simulink model "mpc_blueboat"  (R2024a)
settings: Solver=VariableStepAuto  StartTime=0.0  StopTime=20  RelTol=1e-3
libraries: sharedutil x6, aerolibutil x1, mpclib x1
settings Model: Creator=cdsouza
settings SolverCC: AlgebraicLoopSolver=TrustRegion
settings DataIOCC: ReturnWorkspaceOutputs=off
settings DebuggingCC: UnconnectedInputMsg=warning  UnconnectedOutputMsg=warning  UnconnectedLineMsg=warning  ArithmeticOperatorsInVariantConditions=warning
settings ModelReferenceCC: EnableRefExpFcnMdlSchedulingChecks=on
settings SFSimCC: CustomCodeUndefinedFunction=UseInterfaceOnly
settings RTWCC: GPUComputeCapability=3.5

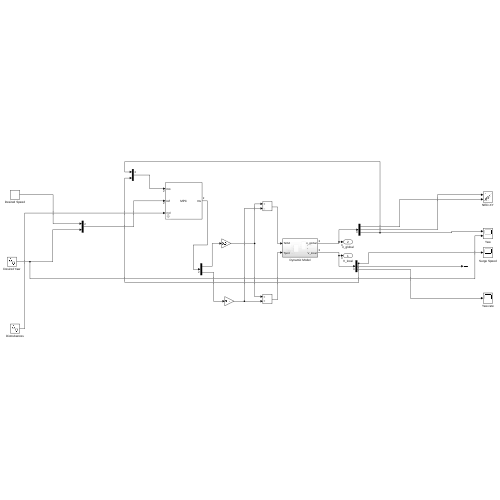
[thumbnail: Simulink's stored preview of the top-level diagram]
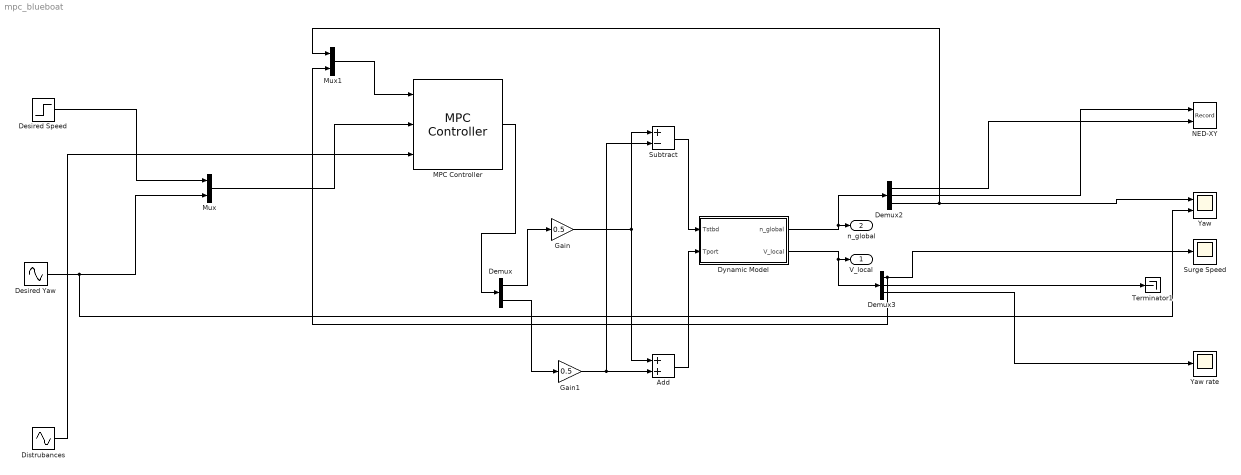
== system mpc_blueboat ==
  Add : Sum
  Demux : Demux  Outputs=2
  Demux2 : Demux  Outputs=3
  Demux3 : Demux  Outputs=3
  Desired Speed : Step  Time=2  SampleTime=0
  Desired Yaw : Sin  Amplitude=5  Frequency=0.5  SampleTime=0
  Distrubances : Sin  Amplitude=0.001  Frequency=0.5  SampleTime=0
  Dynamic Model : Subsystem
  Gain : Gain  Gain=0.5
  Gain1 : Gain  Gain=0.5
  MPC Controller : mpclib/MPC Controller  SCDEnableBlockLinearizationSpecification=on  mpcobj=mpc1  is_multiple=0  enable_value=0  return_u0=off  updateMPCinCallerWorkspace=on  md_inport=on  mv_inport=off  uref_inport=off  return_cost=off  return_mvseq=off  return_qpstatus=off  return_xseq=off  return_state=off  return_ovseq=off  state_inport=off  umin_inport=off  umax_inport=off  ymin_inport=off  ymax_inport=off  cc_inport=off  ywt_inport=off  uwt_inport=off  duwt_inport=off  rhoeps_inport=off  pm_inport=off  MaximumP=10  HorizonChoice=FixedHorizon  n_ts=0.1  n_p=20  n_mv=2  n_md=1  n_ud=0  n_mo=2  n_uo=0  BlockDataType=double  SampleTimeInherited=off  switch_inport=off
  Mux : Mux  Inputs=2
  Mux1 : Mux  Inputs=2
  NED-XY : Record  FileSettingsInternal="{\"entries\":[{\"content\":{\"excelSettings\":{\"content\":{},\"type\":\"Streamout.ExcelSettings\"}},\"type\":\"Streamout.FileSettingStorage\",\"uuid\":\"\"}],\"packageUris\":[\"http:\\/\\/schema.mathworks.com\\/mf0\\/streamout_blocks\\/R2020a\"],\"version\":\"1.0\"}"  Layout=[1 1]  SignalsInternal="{\"entries\":[{\"content\":{\"signals\":[{\"content\":{\"blockPath\":[],\"dimensions\":[1],\"domain\":\"\",\"lineColor\":\"#a2142f\",\"plots\":[ 1 ],\"port\":1,\"sid\":[\"\"],\"signalID\":1,\"signalName\":\"Demux2:2\"},\"type\":\"RecordBlkView.Signal\",\"uuid\":\"\"},{\"content\":{\"blockPath\":[],\"dimensions\":[1],\"domain\":\"\",\"lineColor\":\"#139fff\",\"plots\":[ 1 ],\"port\":2,\"sid\":[\"\"],\"signalID\":2,\"signalName\":\"Demux2:1\"},\"type\":\"RecordBlkView.Signal\",\"uuid\":\"\"},{\"content\":{\"blockPath\":[],\"dimensions\":[3],\"domain\":\"\",\"hasChildren\":true,\"lineColor\":\"#edb120\",\"lineWidth\":2,\"port\":1,\"sid\":[\"\"],\"signalID\":3},\"type\":\"RecordBlkView.Signal\",\"uuid\":\"\"},{\"content\":{\"blockPath\":[],\"channel\":[1],\"dimensions\":[3],\"domain\":\"\",\"lineColor\":\"#b746ff\",\"lineWidth\":2,\"parentID\":3,\"port\":1,\"sid\":[\"\"],\"signalID\":4},\"type\":\"RecordBlkView.Signal\",\"uuid\":\"\"},{\"content\":{\"blockPath\":[],\"dimensions\":[3],\"domain\":\"\",\"hasChildren\":true,\"lineColor\":\"#77ac30\",\"lineWidth\":2,\"port\":1,\"sid\":[\"\"],\"signalID\":5},\"type\":\"RecordBlkView.Signal\",\"uuid\":\"\"},{\"content\":{\"blockPath\":[],\"channel\":[1],\"dimensions\":[3],\"domain\":\"\",\"lineColor\":\"#ff13a6\",\"lineWidth\":2,\"parentID\":5,\"port\":1,\"sid\":[\"\"],\"signalID\":6},\"type\":\"RecordBlkView.Signal\",\"uuid\":\"\"},{\"content\":{\"blockPath\":[],\"dimensions\":[1],\"domain\":\"\",\"hasChildren\":true,\"lineColor\":\"#a2142f\",\"lineWidth\":2,\"port\":1,\"sid\":[\"\"],\"signalID\":7,\"signalName\":\"HydrodynamicCoefficients\"},\"type\":\"RecordBlkView.Signal\",\"uuid\":\"\"},{\"content\":{\"blockPath\":[],\"dimensions\":[1],\"domain\":\"\",\"leafPath\":\"HydrodynamicCoefficients.X_u_dot\",\"lineColor\":\"#139fff\",\"lineWidth\":2,\"parentID\":7,\"port\":1,\"sid\":[\"\"],\"signalID\":8,\"signalName\":\"HydrodynamicCoefficients.X_u_dot\"},\"type\":\"RecordBlkView.Signal\",\"uuid\":\"\"},{\"content\":{\"blockPath\":[],\"dimensions\":[1],\"domain\":\"\",\"leafPath\":\"HydrodynamicCoefficients.Y_v_dot\",\"lineColor\":\"#ff6929\",\"lineWidth\":2,\"parentID\":7,\"port\":1,\"sid\":[\"\"],\"signalID\":9,\"signalName\":\"HydrodynamicCoefficients.Y_v_dot\"},\"type\":\"RecordBlkView.Signal\",\"uuid\":\"\"},{\"content\":{\"blockPath\":[],\"dimensions\":[1],\"domain\":\"\",\"leafPath\":\"HydrodynamicCoefficients.Y_r_dot\",\"lineColor\":\"#b746ff\",\"lineWidth\":2,\"parentID\":7,\"port\":1,\"sid\":[\"\"],\"signalID\":10,\"signalName\":\"HydrodynamicCoefficients.Y_r_dot\"},\"type\":\"RecordBlkView.Signal\",\"uuid\":\"\"},{\"content\":{\"blockPath\":[],\"dimensions\":[1],\"domain\":\"\",\"leafPath\":\"HydrodynamicCoefficients.N_v_dot\",\"lineColor\":\"#64d413\",\"lineWidth\":2,\"parentID\":7,\"port\":1,\"sid\":[\"\"],\"signalID\":11,\"signalName\":\"HydrodynamicCoefficients.N_v_dot\"},\"type\":\"RecordBlkView.Signal\",\"uuid\":\"\"},{\"content\":{\"blockPath\":[],\"dimensions\":[1],\"domain\":\"\",\"leafPath\":\"HydrodynamicCoefficients.N_r_dot\",\"lineColor\":\"#ff13a6\",\"lineWidth\":2,\"parentID\":7,\"port\":1,\"sid\":[\"\"],\"signalID\":12,\"signalName\":\"HydrodynamicCoefficients.N_r_dot\"},\"type\":\"RecordBlkView.Signal\",\"uuid\":\"\"},{\"content\":{\"blockPath\":[],\"dimensions\":[1],\"domain\":\"\",\"leafPath\":\"HydrodynamicCoefficients.X_u\",\"lineColor\":\"#fe330a\",\"lineWidth\":2,\"parentID\":7,\"port\":1,\"sid\":[\"\"],\"signalID\":13,\"signalName\":\"HydrodynamicCoefficients.X_u\"},\"type\":\"RecordBlkView.Signal\",\"uuid\":\"\"},{\"content\":{\"blockPath\":[],\"dimensions\":[1],\"domain\":\"\",\"leafPath\":\"HydrodynamicCoefficients.X_u_u_\",\"lineColor\":\"#22b573\",\"lineWidth\":2,\"parentID\":7,\"port\":1,\"sid\":[\"\"],\"signalID\":14,\"signalName\":\"HydrodynamicCoefficients.X_u_u_\"},\"type\":\"RecordBlkView.Signal\",\"uuid\":\"\"},{\"content\":{\"blockPath\":[],\"dimensions\":[1],\"domain\":\"\",\"leafPath\":\"HydrodynamicCoefficients.Y_v_v_\",\"lineColor\":\"#0072bd\",\"lineWidth\":2,\"parentID\":7,\"port\":1,\"sid\":[\"\"],\"signalID\":15,\"signalName\":\"HydrodynamicCoefficients.Y_v_v_\"},\"type\":\"RecordBlkView.Signal\",\"uuid\":\"\"},{\"content\":{\"blockPath\":[],\"dimensions\":[1],\"domain\":\"\",\"leafPath\":\"HydrodynamicCoefficients.Y_v_r_\",\"lineColor\":\"#d95319\",\"lineWidth\":2,\"parentID\":7,\"port\":1,\"sid\":[\"\"],\"signalID\":16,\"signalName\":\"HydrodynamicCoefficients.Y_v_r_\"},\"type\":\"RecordBlkView.Signal\",\"uuid\":\"\"},{\"content\":{\"blockPath\":[],\"dimensions\":[1],\"domain\":\"\",\"leafPath\":\"HydrodynamicCoefficients.Y_v\",\"lineColor\":\"#edb120\",\"lineWidth\":2,\"parentID\":7,\"port\":1,\"sid\":[\"\"],\"signalID\":17,\"signalName\":\"HydrodynamicCoefficients.Y_v\"},\"type\":\"RecordBlkView.Signal\",\"uuid\":\"\"},{\"content\":{\"blockPath\":[],\"dimensions\":[1],\"domain\":\"\",\"leafPath\":\"HydrodynamicCoefficients.Y_r_v_\",\"lineColor\":\"#7e2f8e\",\"lineWidth\":2,\"parentID\":7,\"port\":1,\"sid\":[\"\"],\"signalID\":18,\"signalName\":\"HydrodynamicCoefficients.Y_r_v_\"},\"type\":\"RecordBlkView.Signal\",\"uuid\":\"\"},{\"content\":{\"blockPath\":[],\"dimensions\":[1],\"domain\":\"\",\"leafPath\":\"HydrodynamicCoefficients.Y_r_r_\",\"lineColor\":\"#77ac30\",\"lineWidth\":2,\"parentID\":7,\"port\":1,\"sid\":[\"\"],\"signalID\":19,\"signalName\":\"HydrodynamicCoefficients.Y_r_r_\"},\"type\":\"RecordBlkView.Signal\",\"uuid\":\"\"},{\"content\":{\"blockPath\":[],\"dimensions\":[1],\"domain\":\"\",\"leafPath\":\"HydrodynamicCoefficients.Y_r\",\"lineColor\":\"#4dbeee\",\"lineWidth\":2,\"parentID\":7,\"port\":1,\"sid\":[\"\"],\"signalID\":20,\"signalName\":\"HydrodynamicCoefficients.Y_r\"},\"type\":\"RecordBlkView.Signal\",\"uuid\":\"\"},{\"content\":{\"blockPath\":[],\"dimensions\":[1],\"domain\":\"\",\"leafPath\":\"HydrodynamicCoefficients.N_v_v_\",\"lineColor\":\"#a2142f\",\"lineWidth\":2,\"parentID\":7,\"port\":1,\"sid\":[\"\"],\"signalID\":21,\"signalName\":\"HydrodynamicCoefficients.N_v_v_\"},\"type\":\"RecordBlkView.Signal\",\"uuid\":\"\"},{\"content\":{\"blockPath\":[],\"dimensions\":[1],\"domain\":\"\",\"leafPath\":\"HydrodynamicCoefficients.N_v\",\"lineColor\":\"#139fff\",\"lineWidth\":2,\"parentID\":7,\"port\":1,\"sid\":[\"\"],\"signalID\":22,\"signalName\":\"HydrodynamicCoefficients.N_v\"},\"type\":\"RecordBlkView.Signal\",\"uuid\":\"\"},{\"content\":{\"blockPath\":[],\"dimensions\":[1],\"domain\":\"\",\"leafPath\":\"HydrodynamicCoefficients.N_v_r_\",\"lineColor\":\"#ff6929\",\"lineWidth\":2,\"parentID\":7,\"port\":1,\"sid\":[\"\"],\"signalID\":23,\"signalName\":\"HydrodynamicCoefficients.N_v_r_\"},\"type\":\"RecordBlkView.Signal\",\"uuid\":\"\"},{\"content\":{\"blockPath\":[],\"dimensions\":[1],\"domain\":\"\",\"leafPath\":\"HydrodynamicCoefficients.N_r_v_\",\"lineColor\":\"#b746ff\",\"lineWidth\":2,\"parentID\":7,\"port\":1,\"sid\":[\"\"],\"signalID\":24,\"signalName\":\"HydrodynamicCoefficients.N_r_v_\"},\"type\":\"RecordBlkView.Signal\",\"uuid\":\"\"},{\"content\":{\"blockPath\":[],\"dimensions\":[1],\"domain\":\"\",\"leafPath\":\"HydrodynamicCoefficients.N_r\",\"lineColor\":\"#64d413\",\"lineWidth\":2,\"parentID\":7,\"port\":1,\"sid\":[\"\"],\"signalID\":25,\"signalName\":\"HydrodynamicCoefficients.N_r\"},\"type\":\"RecordBlkView.Signal\",\"uuid\":\"\"},{\"content\":{\"blockPath\":[],\"dimensions\":[1],\"domain\":\"\",\"leafPath\":\"HydrodynamicCoefficients.N_r_r_\",\"lineColor\":\"#ff13a6\",\"lineWidth\":2,\"parentID\":7,\"port\":1,\"sid\":[\"\"],\"signalID\":26,\"signalName\":\"HydrodynamicCoefficients.N_r_r_\"},\"type\":\"RecordBlkView.Signal\",\"uuid\":\"\"},{\"content\":{\"blockPath\":[],\"channel\":[2],\"dimensions\":[3],\"domain\":\"\",\"lineColor\":\"#edb120\",\"lineWidth\":2,\"parentID\":3,\"port\":1,\"sid\":[\"\"],\"signalID\":27},\"type\":\"RecordBlkView.Signal\",\"uuid\":\"\"},{\"content\":{\"blockPath\":[],\"channel\":[3],\"dimensions\":[3],\"domain\":\"\",\"lineColor\":\"#7e2f8e\",\"lineWidth\":2,\"parentID\":3,\"port\":1,\"sid\":[\"\"],\"signalID\":28},\"type\":\"RecordBlkView.Signal\",\"uuid\":\"\"},{\"content\":{\"blockPath\":[],\"channel\":[2],\"dimensions\":[3],\"domain\":\"\",\"lineColor\":\"#77ac30\",\"lineWidth\":2,\"parentID\":5,\"port\":1,\"sid\":[\"\"],\"signalID\":29},\"type\":\"RecordBlkView.Signal\",\"uuid\":\"\"},{\"content\":{\"blockPath\":[],\"channel\":[3],\"dimensions\":[3],\"domain\":\"\",\"lineColor\":\"#4dbeee\",\"lineWidth\":2,\"parentID\":5,\"port\":1,\"sid\":[\"\"],\"signalID\":30},\"type\":\"RecordBlkView.Signal\",\"uuid\":\"\"}]},\"type\":\"RecordBlkView.InputSignals\",\"uuid\":\"\"}],\"packageUris\":[\"http:\\/\\/schema.mathworks.com\\/mf0\\/streamout_blocks\\/R2020a\"],\"version\":\"1.0\"}"  VisualizationBindings="{\"xyplotplugin\":{\"info\":[{\"series\":[{\"bindingParametersList\":[{\"parameter\":\"X-Axis\",\"signalID\":1,\"signalName\":\"Demux2:2\"},{\"parameter\":\"Y-Axis\",\"signalID\":2,\"signalName\":\"Demux2:1\"}],\"seriesID\":0}],\"subplotID\":1}]}}"  CompatibilityTag=XY  st=-1
  Subtract : Sum  Inputs=+-
  Surge Speed : Scope
  Terminator1 : Terminator
  Yaw : Scope  NumInputPorts=2
  Yaw rate : Scope
  V_local : Outport  VectorParamsAs1DForOutWhenUnconnected=off
  n_global : Outport  Port=2  VectorParamsAs1DForOutWhenUnconnected=off
  wires:
  Dynamic Model/1(n_global) -> Demux2/1, n_global/1
  Demux2/2 -> NED-XY/1
  Demux2/1 -> NED-XY/2
  Demux3/1 -> Mux1/2, Surge Speed/1
  Demux3/3 -> Yaw rate/1
  Dynamic Model/2(V_local) -> Demux3/1, V_local/1
  Demux2/3 -> Mux1/1, Yaw/1
  Demux3/2 -> Terminator1/1
  Desired Yaw/1 -> Yaw/2, Mux/2
  Gain/1 -> Subtract/1, Add/1
  Gain1/1 -> Add/2, Subtract/2
  Add/1 -> Dynamic Model/2(Tport)
  Subtract/1 -> Dynamic Model/1(Tstbd)
  Desired Speed/1 -> Mux/1
  Mux/1 -> MPC Controller/2
  Distrubances/1 -> MPC Controller/3
  Demux/2 -> Gain1/1
  Demux/1 -> Gain/1
  MPC Controller/1 -> Demux/1
  Mux1/1 -> MPC Controller/1

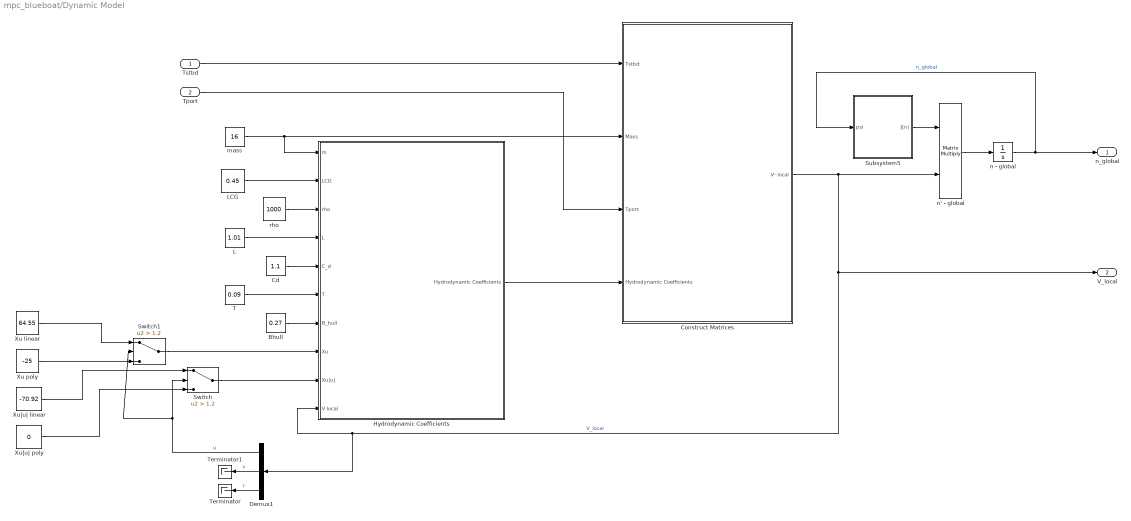
== system mpc_blueboat/Dynamic Model ==
  Tstbd : Inport
  Tport : Inport  Port=2
  "Bhull " : Constant  Value=0.27
  Cd : Constant  Value=1.1
  Construct Matrices : Subsystem
  Demux1 : Demux  Outputs=3
  Hydrodynamic Coefficients : Subsystem
  L : Constant  Value=1.01
  LCG : Constant  Value=0.45
  Subsystem5 : Subsystem
  Switch : Switch  Criteria=u2 > Threshold  Threshold=1.2  SaturateOnIntegerOverflow=off  InputSameDT=off
  Switch1 : Switch  Criteria=u2 > Threshold  Threshold=1.2  SaturateOnIntegerOverflow=off  InputSameDT=off
  T : Constant  Value=0.09
  Terminator : Terminator
  Terminator1 : Terminator
  Xu linear : Constant  Value=64.55
  Xu poly : Constant  Value=-25
  Xu|u| linear : Constant  Value=-70.92
  Xu|u| poly : Constant  Value=0
  mass : Constant  Value=16
  n - global : Integrator  InitialCondition=[0 0 0]
  n' - global : Product  Multiplication=Matrix(*)
  rho : Constant  Value=1000
  n_global : Outport  VectorParamsAs1DForOutWhenUnconnected=off
  V_local : Outport  Port=2  VectorParamsAs1DForOutWhenUnconnected=off
  wires:
  n - global/1 -> n_global/1, Subsystem5/1(psi)  "n_global"
  Cd/1 -> Hydrodynamic Coefficients/5(C_d)
  Construct Matrices/1(V- local) -> Demux1/1, Hydrodynamic Coefficients/10(V local), V_local/1, n' - global/2  "V_local"
  n' - global/1 -> n - global/1
  Subsystem5/1(J(n)) -> n' - global/1
  rho/1 -> Hydrodynamic Coefficients/3(rho)
  L/1 -> Hydrodynamic Coefficients/4(L)
  Tport/1 -> Construct Matrices/3(Tport)
  Tstbd/1 -> Construct Matrices/1(Tstbd)
  mass/1 -> Hydrodynamic Coefficients/1(m), Construct Matrices/2("Mass ")
  Hydrodynamic Coefficients/1("Hydrodynamic Coefficients ") -> Construct Matrices/4(Hydrodynamic Coefficients)
  T/1 -> Hydrodynamic Coefficients/6(T)
  "Bhull "/1 -> Hydrodynamic Coefficients/7(B_hull)
  Switch/1 -> Hydrodynamic Coefficients/9(Xu|u|)
  LCG/1 -> Hydrodynamic Coefficients/2(LCG)
  Demux1/1 -> Switch1/2, Switch/2  "u"
  Xu|u| poly/1 -> Switch/3
  Xu|u| linear/1 -> Switch/1
  Switch1/1 -> Hydrodynamic Coefficients/8(Xu)
  Xu poly/1 -> Switch1/3
  Xu linear/1 -> Switch1/1
  Demux1/3 -> Terminator/1  "r"
  Demux1/2 -> Terminator1/1  "v"

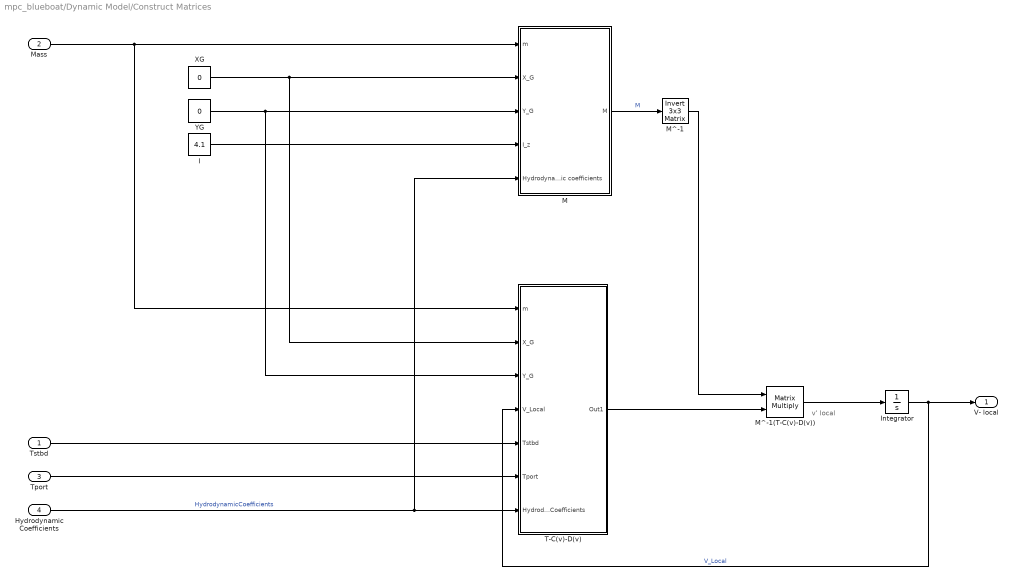
== system mpc_blueboat/Dynamic Model/Construct Matrices ==
  note: v' local
  Tstbd : Inport
  "Mass " : Inport  Port=2
  Tport : Inport  Port=3
  Hydrodynamic Coefficients : Inport  Port=4
  I : Constant  Value=4.1
  Integrator : Integrator
  M : Subsystem
  M^-1 : aerolibutil/Invert  3x3 Matrix
  M^-1(T-C(v)-D(v)) : Product  Multiplication=Matrix(*)
  T-C(v)-D(v) : Subsystem
  XG : Constant  Value=0
  YG : Constant  Value=0
  V- local : Outport  VectorParamsAs1DForOutWhenUnconnected=off
  wires:
  M/1(M) -> M^-1/1  "M"
  Integrator/1 -> V- local/1, T-C(v)-D(v)/4(V_Local)  "V_Local"
  M^-1(T-C(v)-D(v))/1 -> Integrator/1
  I/1 -> M/4(I_z)
  M^-1/1 -> M^-1(T-C(v)-D(v))/1
  Hydrodynamic Coefficients/1 -> M/5(Hydrodynamic coefficients), T-C(v)-D(v)/7(HydrodynamicCoefficients)  "HydrodynamicCoefficients"
  YG/1 -> T-C(v)-D(v)/3(Y_G), M/3(Y_G)
  "Mass "/1 -> T-C(v)-D(v)/1(m), M/1(m)
  XG/1 -> T-C(v)-D(v)/2(X_G), M/2(X_G)
  Tstbd/1 -> T-C(v)-D(v)/5(Tstbd)
  Tport/1 -> T-C(v)-D(v)/6(Tport)
  T-C(v)-D(v)/1(Out1) -> M^-1(T-C(v)-D(v))/2

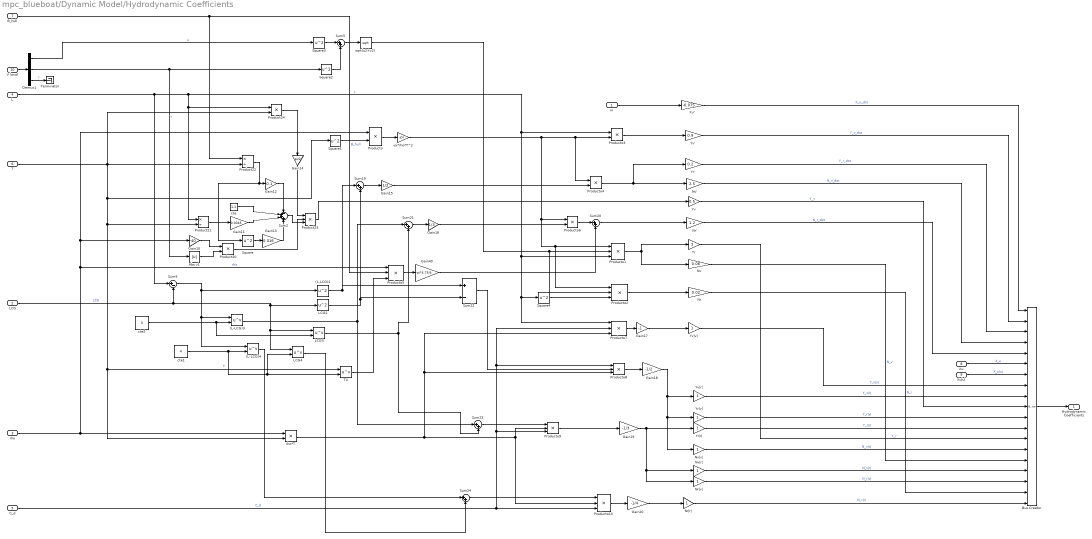
== system mpc_blueboat/Dynamic Model/Hydrodynamic Coefficients ==
  m : Inport
  LCG : Inport  Port=2
  rho : Inport  Port=3
  L : Inport  Port=4
  C_d : Inport  Port=5
  T : Inport  Port=6
  B_hull : Inport  Port=7
  Xu : Inport  Port=8
  Xu|u| : Inport  Port=9
  V local : Inport  Port=10
  (L-LCG)2 : Math  Operator=square  SignedPower=on
  (L-LCG)3 : Math  Operator=pow  SignedPower=on
  (L-LCG)4 : Math  Operator=pow  SignedPower=on
  -pi*rho*T^2 : Gain  Gain=-pi
  Abs v1 : Abs  SaturateOnIntegerOverflow=off
  Bus Creator : BusCreator  Inputs=19
  Demux1 : Demux  Outputs=3
  Gain10 : Gain  Gain=-40
  Gain11 : Gain  Gain=0.0045
  Gain12 : Gain  Gain=0.1
  Gain13 : Gain  Gain=0.016
  Gain14 : Gain  Gain=pi/2
  Gain15 : Gain  Gain=1/2
  Gain16 : Gain  Gain=1/3
  Gain17 : Gain  Gain=-1
  Gain18 : Gain  Gain=-1/2
  Gain19 : Gain  Gain=-1/3
  Gain20 : Gain  Gain=-1/4
  Gain40 : Gain  Gain=-pi*4.75/4
  LCG2 : Math  Operator=square  SignedPower=on
  LCG3 : Math  Operator=pow  SignedPower=on
  LCG4 : Math  Operator=pow  SignedPower=on
  Nr : Gain  Gain=0.02
  Nr' : Gain  Gain=1.2
  Nr|r| : Gain
  Nr|v| : Gain
  Nv : Gain  Gain=0.06
  Nv' : Gain  Gain=2.5
  Nv|r| : Gain
  Nv|v| : Gain
  Product20 : Product
  Product21 : Product  Inputs=*/
  Product22 : Product  Inputs=*/
  Product23 : Product  Inputs=3
  Product24 : Product
  Producto{,3..4,6} (4 alike) : Product
  Producto{1..2,5,7..10} (7 alike) : Product  Inputs=3
  Square{,1..4} (5 alike) : Math  Operator=square  SignedPower=on
  Sum{5,19..21,23..24} (6 alike) : Sum  Inputs=|++
  Sum2 : Sum  Inputs=-+++
  Sum22 : Sum  Inputs=|+-
  Sum9 : Sum  Inputs=|+-
  T4 : Math  Operator=pow  SignedPower=on
  Terminator : Terminator
  Xu' : Gain  Gain=-0.075
  Yr : Gain  Gain=3
  Yr' : Gain  Gain=0.2
  Yr|r| : Gain
  Yr|v| : Gain
  Yv : Gain  Gain=0.5
  Yv' : Gain  Gain=0.9
  Yv|r| : Gain
  Yv|v| : Gain
  cte : Constant  Value=1.1
  cte1 : Constant  Value=4
  cte2 : Constant  Value=3
  rho*T : Product
  sqrt(u2+v2) : Sqrt
  "Hydrodynamic Coefficients " : Outport  VectorParamsAs1DForOutWhenUnconnected=off
  wires:
  m/1 -> Xu'/1
  Nv'/1 -> Bus Creator/4  "N_v_dot"
  Xu'/1 -> Bus Creator/1  "X_u_dot"
  Square/1 -> Gain13/1
  Gain14/1 -> Product23/1
  Product24/1 -> Gain14/1
  Sum9/1 -> (L-LCG)3/1, (L-LCG)4/1, (L-LCG)2/1
  Square4/1 -> Producto2/3
  sqrt(u2+v2)/1 -> Producto2/2, Producto1/2
  Product20/1 -> Product23/2
  Gain13/1 -> Sum2/4
  B_hull/1 -> Producto5/2, Product22/1  "B_hull"
  Square2/1 -> Sum5/2
  Sum20/1 -> Nr'/1
  Gain12/1 -> Sum2/1
  Sum21/1 -> Gain16/1
  LCG4/1 -> Sum24/2
  Sum24/1 -> Producto10/1
  (L-LCG)4/1 -> Sum24/1
  Sum2/1 -> Product23/3
  Producto10/1 -> Gain20/1
  (L-LCG)3/1 -> Sum21/1, Sum23/1
  Producto6/1 -> Sum20/1
  Gain19/1 -> Yr|r|/1, Nr|v|/1, Nv|r|/1
  Gain16/1 -> Producto6/2
  Sum22/1 -> Producto8/2
  Producto3/1 -> Yv'/1
  Gain10/1 -> Product20/1
  cte1/1 -> LCG4/2, T4/2, (L-LCG)4/2
  cte2/1 -> (L-LCG)3/2, LCG3/2
  Product23/1 -> Yv/1
  cte/1 -> Sum2/2
  Producto8/1 -> Gain18/1
  Sum23/1 -> Producto9/1
  Gain20/1 -> Nr|r|/1
  Gain18/1 -> Nv|v|/1, Yr|v|/1, Yv|r|/1
  Yr'/1 -> Bus Creator/3  "Y_r_dot"
  Producto7/1 -> Gain17/1
  Producto9/1 -> Gain19/1
  Gain11/1 -> Sum2/3
  Square1/1 -> Producto/2
  Producto2/1 -> Nr/1
  LCG3/1 -> Sum21/2, Sum23/2
  T4/1 -> Producto5/3
  Gain40/1 -> Sum20/2
  Producto4/1 -> Yr'/1, Nv'/1
  Sum19/1 -> Gain15/1
  Square3/1 -> Sum5/1
  Sum5/1 -> sqrt(u2+v2)/1
  rho/1 -> Producto/1, Gain10/1, Producto5/1, rho*T/1  "rho"
  Abs v1/1 -> Product20/2
  Product21/1 -> Gain11/1
  Gain17/1 -> Yv|v|/1
  (L-LCG)2/1 -> Sum19/1, Sum22/1
  Producto1/1 -> Nv/1, Yr/1
  Product22/1 -> Square/1, Gain12/1
  LCG2/1 -> Sum19/2, Sum22/2
  LCG/1 -> Sum9/2, LCG2/1, LCG3/1, LCG4/1  "LCG"
  Producto/1 -> -pi*rho*T^2/1
  -pi*rho*T^2/1 -> Producto4/1, Producto3/2, Producto2/1, Producto1/1, Producto6/1
  Producto5/1 -> Gain40/1
  Gain15/1 -> Producto4/2
  rho*T/1 -> Producto9/2, Producto10/2, Producto7/3, Producto8/3
  T/1 -> Product21/2, rho*T/2, T4/1, Square1/1, Product22/2, Product24/2  "T"
  L/1 -> Producto7/1, Square4/1, Producto1/3, Producto3/1, Product21/1, Product24/1, Sum9/1  "L"
  C_d/1 -> Producto7/2, Producto8/1, Producto9/3, Producto10/3  "C_d"
  Nv/1 -> Bus Creator/15  "N_v"
  Yv|v|/1 -> Bus Creator/8  "Y_v|v|"
  Yr|r|/1 -> Bus Creator/12  "Y_r|r|"
  Yv/1 -> Bus Creator/10  "Y_v"
  Nv|v|/1 -> Bus Creator/14  "N_v|v|"
  Yr|v|/1 -> Bus Creator/11  "Y_r|v|"
  Nv|r|/1 -> Bus Creator/16  "N_v|r|"
  Yr/1 -> Bus Creator/13  "Y_r"
  Nr|r|/1 -> Bus Creator/19  "N_r|r|"
  Nr/1 -> Bus Creator/18  "N_r"
  Xu|u|/1 -> Bus Creator/7  "X_u|u|"
  Yv|r|/1 -> Bus Creator/9  "Y_v|r|"
  Nr|v|/1 -> Bus Creator/17  "N_r|v|"
  Xu/1 -> Bus Creator/6  "X_u"
  Bus Creator/1 -> "Hydrodynamic Coefficients "/1
  Nr'/1 -> Bus Creator/5  "N_r_dot"
  Yv'/1 -> Bus Creator/2  "Y_v_dot"
  Demux1/1 -> Square3/1  "u"
  V local/1 -> Demux1/1
  Demux1/2 -> Abs v1/1, Square2/1  "v"
  Demux1/3 -> Terminator/1  "r"

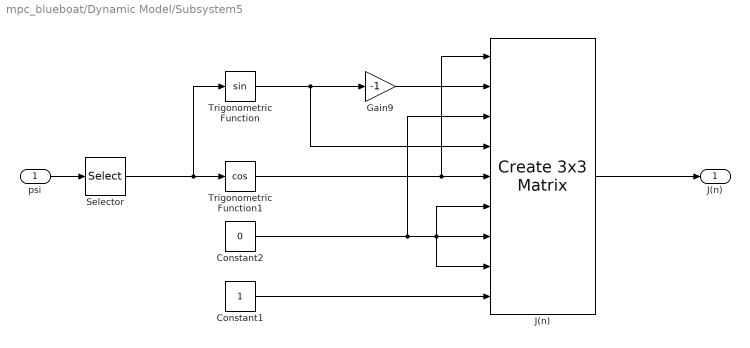
== system mpc_blueboat/Dynamic Model/Subsystem5 ==
  psi : Inport
  " J(n)" : sharedutil/Create 3x3 Matrix  aMode=aMode
  Constant1 : Constant
  Constant2 : Constant  Value=0
  Gain9 : Gain  Gain=-1
  Selector : Selector  InputPortWidth=3  IndexOptions=Index vector (dialog)  Indices=3  OutputSizes=1
  Trigonometric Function : Trigonometry
  Trigonometric Function1 : Trigonometry  Operator=cos
  J(n) : Outport  VectorParamsAs1DForOutWhenUnconnected=off
  wires:
  Gain9/1 -> " J(n)"/2
  Trigonometric Function1/1 -> " J(n)"/5, " J(n)"/1
  Trigonometric Function/1 -> " J(n)"/4, Gain9/1
  Constant1/1 -> " J(n)"/9
  psi/1 -> Selector/1
  " J(n)"/1 -> J(n)/1
  Constant2/1 -> " J(n)"/8, " J(n)"/7, " J(n)"/6, " J(n)"/3
  Selector/1 -> Trigonometric Function1/1, Trigonometric Function/1

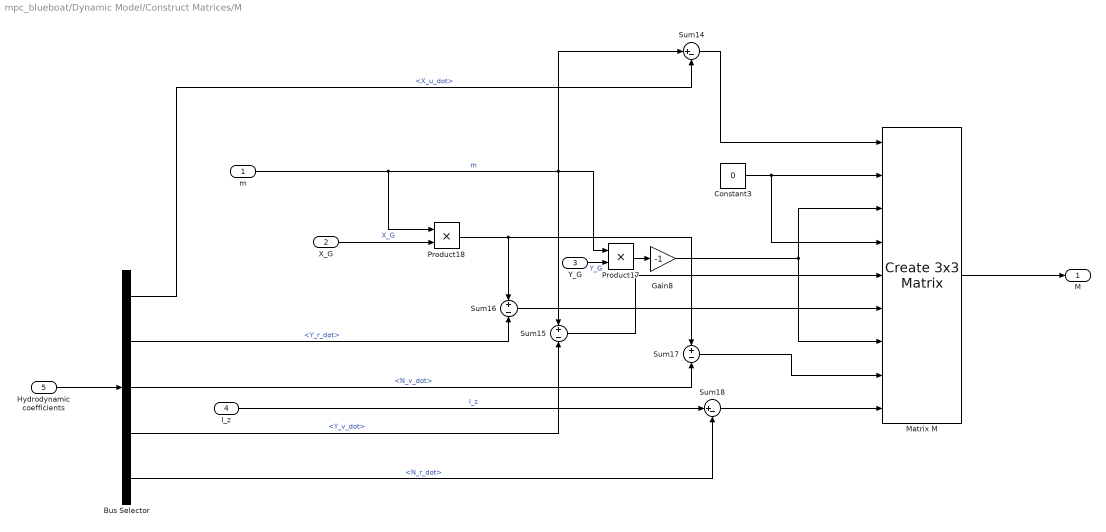
== system mpc_blueboat/Dynamic Model/Construct Matrices/M ==
  m : Inport
  X_G : Inport  Port=2
  Y_G : Inport  Port=3
  I_z : Inport  Port=4
  Hydrodynamic coefficients : Inport  Port=5
  Bus Selector : BusSelector  OutputSignals=X_u_dot,Y_r_dot,N_v_dot,Y_v_dot,N_r_dot
  Constant3 : Constant  Value=0
  Gain8 : Gain  Gain=-1
  Matrix M : sharedutil/Create 3x3 Matrix  aMode=aMode
  Product17 : Product
  Product18 : Product
  Sum14 : Sum  Inputs=|+-
  Sum15 : Sum  Inputs=+-
  Sum16 : Sum  Inputs=+-
  Sum17 : Sum  Inputs=+-
  Sum18 : Sum  Inputs=|+-
  M : Outport  VectorParamsAs1DForOutWhenUnconnected=off
  wires:
  Gain8/1 -> Matrix M/7, Matrix M/3
  Product17/1 -> Gain8/1
  Product18/1 -> Sum17/1, Sum16/1
  Sum18/1 -> Matrix M/9
  Constant3/1 -> Matrix M/4, Matrix M/2
  I_z/1 -> Sum18/1  "I_z"
  Sum15/1 -> Matrix M/5
  m/1 -> Sum14/1, Product17/1, Sum15/1, Product18/1  "m"
  Bus Selector/3 -> Sum17/2  "<N_v_dot>"
  Sum14/1 -> Matrix M/1
  Sum16/1 -> Matrix M/6
  Matrix M/1 -> M/1
  Sum17/1 -> Matrix M/8
  X_G/1 -> Product18/2  "X_G"
  Y_G/1 -> Product17/2  "Y_G"
  Bus Selector/1 -> Sum14/2  "<X_u_dot>"
  Hydrodynamic coefficients/1 -> Bus Selector/1
  Bus Selector/2 -> Sum16/2  "<Y_r_dot>"
  Bus Selector/4 -> Sum15/2  "<Y_v_dot>"
  Bus Selector/5 -> Sum18/2  "<N_r_dot>"

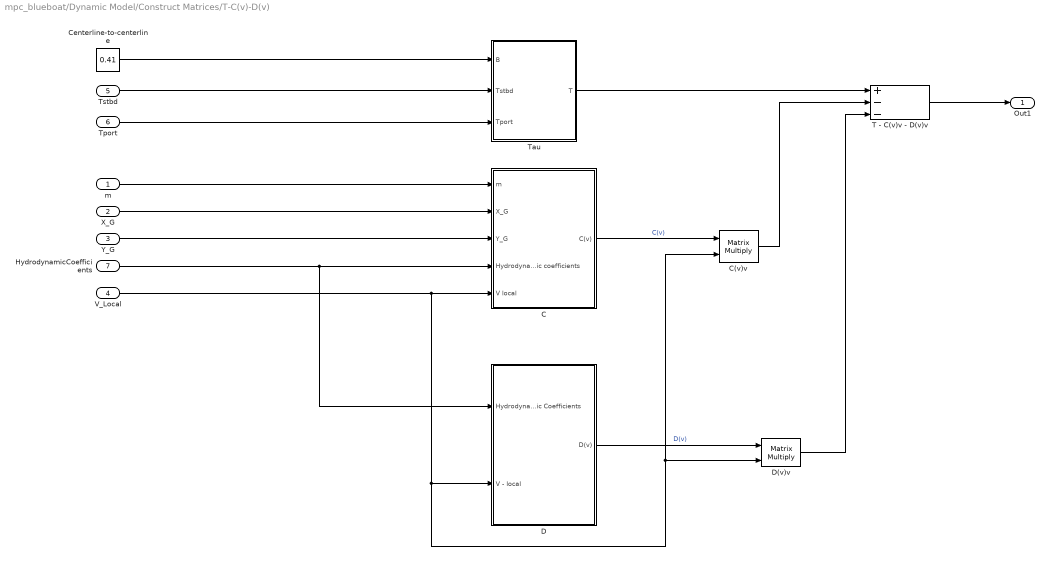
== system mpc_blueboat/Dynamic Model/Construct Matrices/T-C(v)-D(v) ==
  m : Inport
  X_G : Inport  Port=2
  Y_G : Inport  Port=3
  V_Local : Inport  Port=4
  Tstbd : Inport  Port=5
  Tport : Inport  Port=6
  HydrodynamicCoefficients : Inport  Port=7
  C : Subsystem
  C(v)v : Product  Multiplication=Matrix(*)
  Centerline-to-centerline : Constant  Value=0.41
  D : Subsystem
  D(v)v : Product  Multiplication=Matrix(*)
  T - C(v)v - D(v)v : Sum  Inputs=+--
  Tau : Subsystem
  Out1 : Outport  VectorParamsAs1DForOutWhenUnconnected=off
  wires:
  Tstbd/1 -> Tau/2(Tstbd)
  V_Local/1 -> D(v)v/2, C(v)v/2, D/2(V - local), C/5(V local)
  T - C(v)v - D(v)v/1 -> Out1/1
  D(v)v/1 -> T - C(v)v - D(v)v/3
  C(v)v/1 -> T - C(v)v - D(v)v/2
  Centerline-to-centerline/1 -> Tau/1(B)
  C/1(C(v)) -> C(v)v/1  "C(v)"
  Tport/1 -> Tau/3(Tport)
  Tau/1(T) -> T - C(v)v - D(v)v/1
  D/1(D(v)) -> D(v)v/1  "D(v)"
  HydrodynamicCoefficients/1 -> C/4(Hydrodynamic coefficients), D/1(Hydrodynamic Coefficients)
  Y_G/1 -> C/3(Y_G)
  X_G/1 -> C/2(X_G)
  m/1 -> C/1(m)

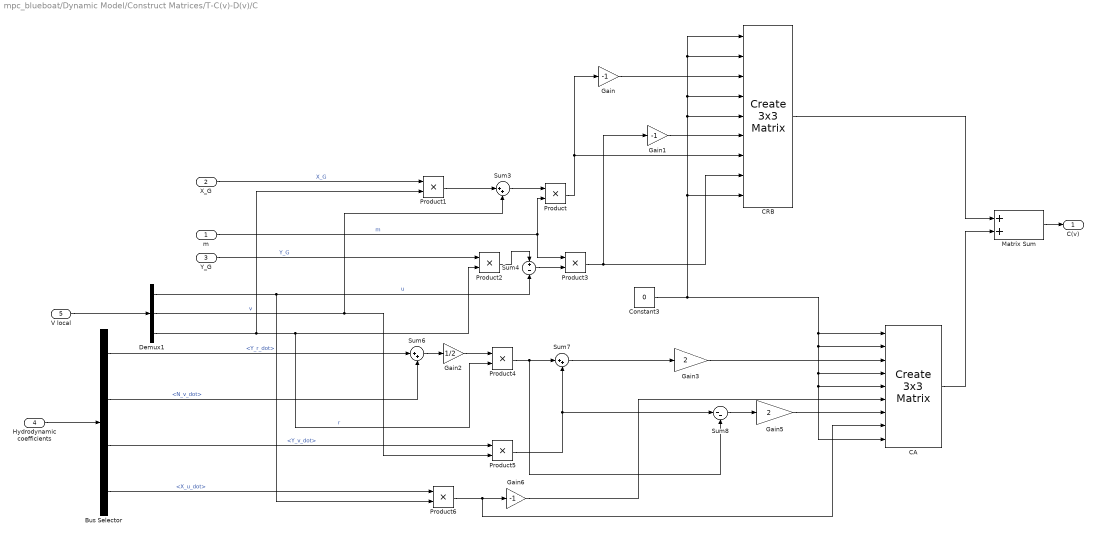
== system mpc_blueboat/Dynamic Model/Construct Matrices/T-C(v)-D(v)/C ==
  m : Inport
  X_G : Inport  Port=2
  Y_G : Inport  Port=3
  Hydrodynamic coefficients : Inport  Port=4
  V local : Inport  Port=5
  " CRB" : sharedutil/Create 3x3 Matrix  aMode=aMode
  Bus Selector : BusSelector  OutputSignals=Y_r_dot,N_v_dot,Y_v_dot,X_u_dot
  CA : sharedutil/Create 3x3 Matrix  aMode=aMode
  Constant3 : Constant  Value=0
  Demux1 : Demux  Outputs=3
  Gain : Gain  Gain=-1
  Gain1 : Gain  Gain=-1
  Gain2 : Gain  Gain=1/2
  Gain3 : Gain  Gain=2
  Gain5 : Gain  Gain=2
  Gain6 : Gain  Gain=-1
  Matrix Sum : Sum
  Product{,1..6} (7 alike) : Product
  Sum3 : Sum  Inputs=|++
  Sum4 : Sum  Inputs=+-
  Sum6 : Sum  Inputs=|++
  Sum7 : Sum  Inputs=|++
  Sum8 : Sum  Inputs=|--
  C(v) : Outport  VectorParamsAs1DForOutWhenUnconnected=off
  wires:
  Bus Selector/1 -> Sum6/1  "<Y_r_dot>"
  Demux1/3 -> Product1/2, Product2/2, Product4/2  "r"
  Gain2/1 -> Product4/1
  CA/1 -> Matrix Sum/2
  Gain/1 -> " CRB"/3
  Bus Selector/2 -> Sum6/2  "<N_v_dot>"
  Sum3/1 -> Product/1
  Sum8/1 -> Gain5/1
  Product2/1 -> Sum4/1
  Sum6/1 -> Gain2/1
  Product5/1 -> Sum7/2, Sum8/1
  Gain1/1 -> " CRB"/6
  Product1/1 -> Sum3/1
  Y_G/1 -> Product2/1  "Y_G"
  Matrix Sum/1 -> C(v)/1
  Gain3/1 -> CA/3
  Gain6/1 -> CA/6
  Product6/1 -> Gain6/1, CA/8
  Demux1/2 -> Sum3/2, Product5/2  "v"
  Product4/1 -> Sum7/1, Sum8/2
  Product3/1 -> " CRB"/8, Gain1/1
  Gain5/1 -> CA/7
  " CRB"/1 -> Matrix Sum/1
  X_G/1 -> Product1/1  "X_G"
  Sum7/1 -> Gain3/1
  Product/1 -> " CRB"/7, Gain/1
  m/1 -> Product/2, Product3/1  "m"
  Constant3/1 -> " CRB"/5, " CRB"/4, " CRB"/2, " CRB"/1, " CRB"/9, CA/4, CA/5, CA/9, CA/2, CA/1
  Hydrodynamic coefficients/1 -> Bus Selector/1
  Bus Selector/4 -> Product6/1  "<X_u_dot>"
  Bus Selector/3 -> Product5/1  "<Y_v_dot>"
  Demux1/1 -> Sum4/2, Product6/2  "u"
  V local/1 -> Demux1/1
  Sum4/1 -> Product3/2

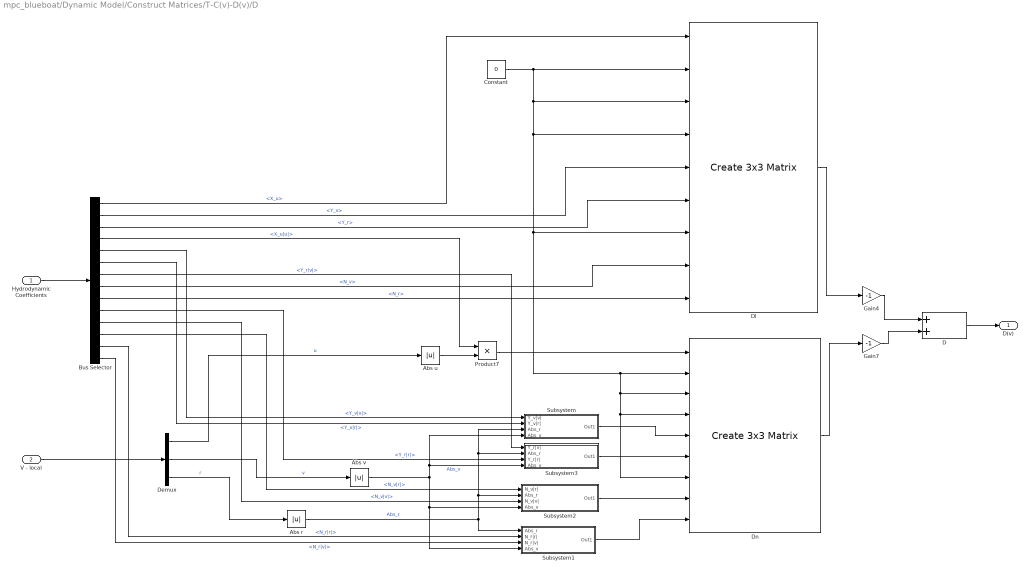
== system mpc_blueboat/Dynamic Model/Construct Matrices/T-C(v)-D(v)/D ==
  Hydrodynamic Coefficients : Inport
  V - local : Inport  Port=2
  Abs r : Abs  SaturateOnIntegerOverflow=off
  Abs u : Abs  SaturateOnIntegerOverflow=off
  Abs v : Abs  SaturateOnIntegerOverflow=off
  Bus Selector : BusSelector  OutputSignals=X_u,Y_v,Y_r,X_u|u|,Y_v|v|,Y_v|r|,Y_r|v|,N_v,N_r,Y_r|r|,N_v|v|,N_v|r|,N_r|r|,N_r|v|
  Constant : Constant  Value=0
  D : Sum
  Demux : Demux  Outputs=3
  Dl : sharedutil/Create 3x3 Matrix  aMode=aMode
  Dn : sharedutil/Create 3x3 Matrix  aMode=aMode
  Gain4 : Gain  Gain=-1
  Gain7 : Gain  Gain=-1
  Product7 : Product
  Subsystem : Subsystem
  Subsystem1 : Subsystem
  Subsystem2 : Subsystem
  Subsystem3 : Subsystem
  D(v) : Outport  VectorParamsAs1DForOutWhenUnconnected=off
  wires:
  Constant/1 -> Dn/7, Dn/4, Dn/3, Dn/2, Dl/7, Dl/4, Dl/3, Dl/2
  Abs u/1 -> Product7/2
  Abs r/1 -> Subsystem/3(Abs_r), Subsystem3/2("Abs_r "), Subsystem2/2(Abs_r), Subsystem1/1(Abs_r)  "Abs_r"
  Product7/1 -> Dn/1
  Abs v/1 -> Subsystem/4("Abs_v "), Subsystem3/4(Abs_v), Subsystem1/4(Abs_v), Subsystem2/4(Abs_v)  "Abs_v"
  Gain7/1 -> D/2
  Gain4/1 -> D/1
  Dl/1 -> Gain4/1
  Dn/1 -> Gain7/1
  D/1 -> D(v)/1
  Subsystem/1(Out1) -> Dn/5
  Subsystem1/1(Out1) -> Dn/9
  Subsystem2/1(Out1) -> Dn/8
  Subsystem3/1(Out1) -> Dn/6
  Hydrodynamic Coefficients/1 -> Bus Selector/1
  Bus Selector/5 -> Subsystem/1("Y_v|v| ")  "<Y_v|v|>"
  Bus Selector/6 -> Subsystem/2(Y_v|r|)  "<Y_v|r|>"
  Bus Selector/2 -> Dl/5  "<Y_v>"
  Bus Selector/7 -> Subsystem3/1(Y_r|v|)  "<Y_r|v|>"
  Bus Selector/10 -> Subsystem3/3(Y_r|r|)  "<Y_r|r|>"
  Bus Selector/11 -> Subsystem2/3(N_v|v|)  "<N_v|v|>"
  Bus Selector/8 -> Dl/8  "<N_v>"
  Bus Selector/12 -> Subsystem2/1(N_v|r|)  "<N_v|r|>"
  Bus Selector/14 -> Subsystem1/3(N_r|v|)  "<N_r|v|>"
  Bus Selector/9 -> Dl/9  "<N_r>"
  Bus Selector/13 -> Subsystem1/2(N_r|r|)  "<N_r|r|>"
  Bus Selector/1 -> Dl/1  "<X_u>"
  Bus Selector/4 -> Product7/1  "<X_u|u|>"
  Bus Selector/3 -> Dl/6  "<Y_r>"
  Demux/1 -> Abs u/1  "u"
  Demux/2 -> Abs v/1  "v"
  Demux/3 -> Abs r/1  "r"
  V - local/1 -> Demux/1

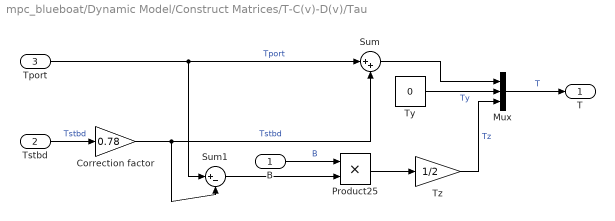
== system mpc_blueboat/Dynamic Model/Construct Matrices/T-C(v)-D(v)/Tau ==
  B : Inport
  Tstbd : Inport  Port=2
  Tport : Inport  Port=3
  Correction factor : Gain  Gain=0.78
  Mux : Mux  Inputs=3
  Product25 : Product
  Sum : Sum  Inputs=|++
  Sum1 : Sum  Inputs=|+-
  Ty : Constant  Value=0
  Tz : Gain  Gain=1/2
  T : Outport  VectorParamsAs1DForOutWhenUnconnected=off
  wires:
  Product25/1 -> Tz/1
  Tz/1 -> Mux/3  "Tz"
  Mux/1 -> T/1  "T"
  B/1 -> Product25/1  "B"
  Sum1/1 -> Product25/2
  Ty/1 -> Mux/2  "Ty"
  Tstbd/1 -> Correction factor/1  "Tstbd"
  Tport/1 -> Sum/1, Sum1/1  "Tport"
  Sum/1 -> Mux/1
  Correction factor/1 -> Sum/2, Sum1/2  "Tstbd"

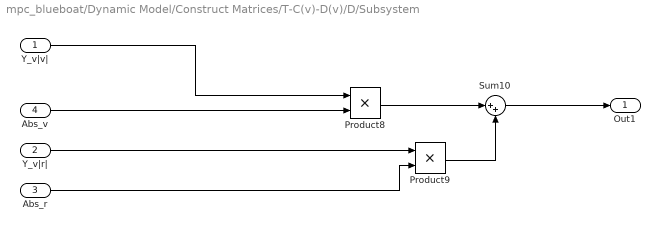
== system mpc_blueboat/Dynamic Model/Construct Matrices/T-C(v)-D(v)/D/Subsystem ==
  "Y_v|v| " : Inport
  Y_v|r| : Inport  Port=2
  Abs_r : Inport  Port=3
  "Abs_v " : Inport  Port=4
  Product8 : Product
  Product9 : Product
  Sum10 : Sum  Inputs=|++
  Out1 : Outport  VectorParamsAs1DForOutWhenUnconnected=off
  wires:
  Y_v|r|/1 -> Product9/1
  Abs_r/1 -> Product9/2
  Product9/1 -> Sum10/2
  "Y_v|v| "/1 -> Product8/1
  Product8/1 -> Sum10/1
  "Abs_v "/1 -> Product8/2
  Sum10/1 -> Out1/1

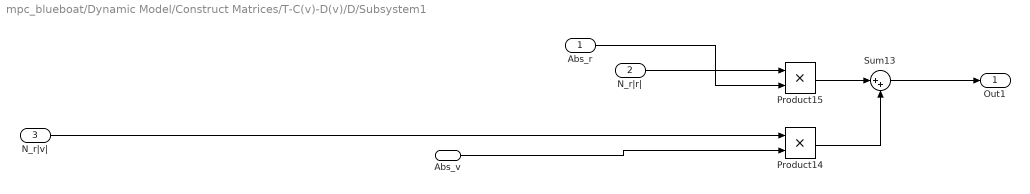
== system mpc_blueboat/Dynamic Model/Construct Matrices/T-C(v)-D(v)/D/Subsystem1 ==
  Abs_r : Inport
  N_r|r| : Inport  Port=2
  N_r|v| : Inport  Port=3
  Abs_v : Inport  Port=4
  Product14 : Product
  Product15 : Product
  Sum13 : Sum  Inputs=|++
  Out1 : Outport  VectorParamsAs1DForOutWhenUnconnected=off
  wires:
  Product15/1 -> Sum13/1
  Sum13/1 -> Out1/1
  N_r|v|/1 -> Product14/1
  Product14/1 -> Sum13/2
  Abs_r/1 -> Product15/2
  N_r|r|/1 -> Product15/1
  Abs_v/1 -> Product14/2

== system mpc_blueboat/Dynamic Model/Construct Matrices/T-C(v)-D(v)/D/Subsystem2 ==
  N_v|r| : Inport
  Abs_r : Inport  Port=2
  N_v|v| : Inport  Port=3
  Abs_v : Inport  Port=4
  Product12 : Product
  Product13 : Product
  Sum12 : Sum  Inputs=|++
  Out1 : Outport  VectorParamsAs1DForOutWhenUnconnected=off
  wires:
  Sum12/1 -> Out1/1
  Product13/1 -> Sum12/1
  N_v|v|/1 -> Product12/1
  Product12/1 -> Sum12/2
  Abs_r/1 -> Product13/2
  Abs_v/1 -> Product12/2
  N_v|r|/1 -> Product13/1

== system mpc_blueboat/Dynamic Model/Construct Matrices/T-C(v)-D(v)/D/Subsystem3 ==
  Y_r|v| : Inport
  "Abs_r " : Inport  Port=2
  Y_r|r| : Inport  Port=3
  Abs_v : Inport  Port=4
  Product10 : Product
  Product11 : Product
  Sum11 : Sum  Inputs=|++
  Out1 : Outport  VectorParamsAs1DForOutWhenUnconnected=off
  wires:
  Product11/1 -> Sum11/2
  Product10/1 -> Sum11/1
  Sum11/1 -> Out1/1
  Y_r|v|/1 -> Product10/1
  "Abs_r "/1 -> Product11/2
  Y_r|r|/1 -> Product11/1
  Abs_v/1 -> Product10/2
